simulink subsystem "Day3_Scenario_1"  (R2024a)
settings: Solver=VariableStepAuto  StartTime=0.0  StopTime=10.0  RelTol=1e-3
undefined symbols (not defined in the file): left_first_line_point_x, right_first_line_point_x
libraries: CarMaker4SL x6, slpidlib x1
settings Model: Creator=junhyung.cha  LastModifiedBy=junhyung.cha

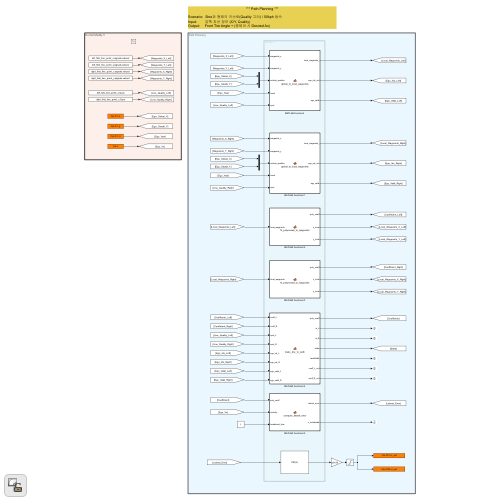
[thumbnail: Simulink's stored preview of the top-level diagram]
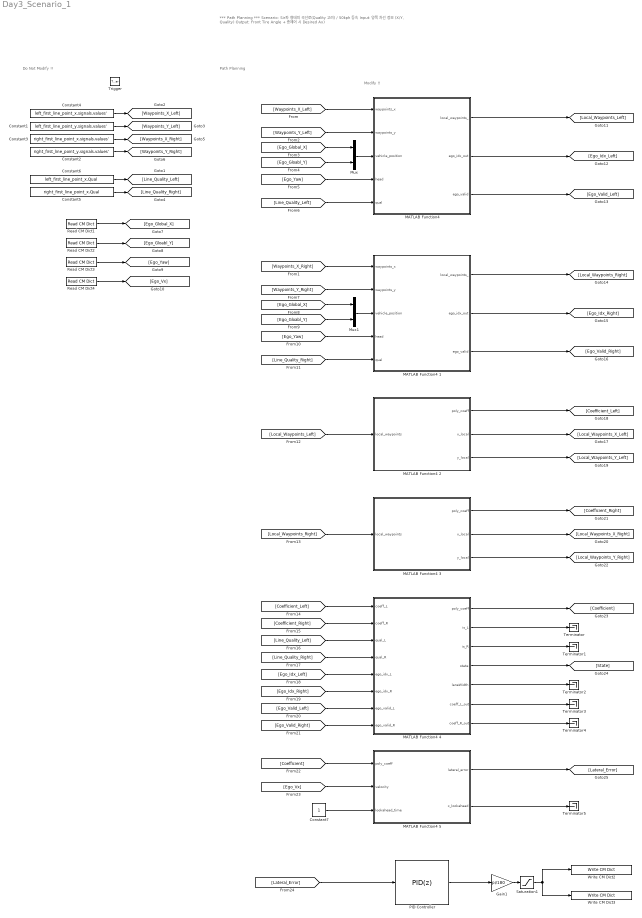
== system Day3_Scenario_1 ==
  note: Path Planning
  note: Do Not Modify !!
  note: Modify !!
  note: *** Path Planning ***
      |
      | Scenario: Sine파 형태의 곡선로(Quality 고려) / 50kph 등속
      | Input: 양쪽 차선 정보 (X/Y, Quality)
      | Output: Front Tire Angle + (종제어 시 Desired Ax)
  Trigger : TriggerPort  TriggerType=function-call  VariantControl=(inherit)
  Constant1 : Constant  Value=left_first_line_point_y.signals.values'
  Constant2 : Constant  Value=right_first_line_point_y.signals.values'
  Constant3 : Constant  Value=right_first_line_point_x.signals.values'
  Constant4 : Constant  Value=left_first_line_point_x.signals.values'
  Constant5 : Constant  Value=right_first_line_point_x.Qual
  Constant6 : Constant  Value=left_first_line_point_x.Qual
  Constant7 : Constant
  Gain1 : Gain  Gain=pi/180
  "MATLAB Function4 " : MATLAB Function  TreatAsAtomicUnit=on
  MATLAB Function4 1 : MATLAB Function  TreatAsAtomicUnit=on
  MATLAB Function4 2 : MATLAB Function  TreatAsAtomicUnit=on
  MATLAB Function4 3 : MATLAB Function  TreatAsAtomicUnit=on
  MATLAB Function4 4 : MATLAB Function  TreatAsAtomicUnit=on
  MATLAB Function4 5 : MATLAB Function  TreatAsAtomicUnit=on
  Mux : Mux  Inputs=2
  Mux1 : Mux  Inputs=2
  PID Controller : slpidlib/PID Controller  Controller=PID  Form=Parallel  TimeDomain=Discrete-time  UseExternalTs=off  SampleTime=-1  IntegratorMethod=Forward Euler  FilterMethod=Forward Euler  ControllerParametersSource=internal  P=3  I=0.01  UseKiTs=off  D=0  UseExternalDerivativeSource=off  N=100  UseFilter=on  TunerSelectOption=Transfer Function Based (PID Tuner App)  InitialConditionSource=internal  InitialConditionForIntegrator=0  InitialConditionForFilter=0  DifferentiatorICPrevScaledInput=0  ExternalReset=none  TrackingMode=off  Kt=1  LimitOutput=off  SatLimitsSource=internal  UpperSaturationLimit=inf  LowerSaturationLimit=-inf  LinearizeAsGain=on  AntiWindupMode=none  Kb=1  LimitIntegrator=off  UpperIntegratorSaturationLimit=inf  LowerIntegratorSaturationLimit=-inf  POutMin=[]  POutMax=[]  IOutMin=[]  IOutMax=[]  DOutMin=[]  DOutMax=[]  NOutMin=[]  NOutMax=[]  SumOutMin=[]  SumOutMax=[]  SaturationOutMin=[]  SaturationOutMax=[]  PParamMin=[]  PParamMax=[]  IParamMin=[]  IParamMax=[]  DParamMin=[]  DParamMax=[]  NParamMin=[]  NParamMax=[]  KbParamMin=[]  KbParamMax=[]  KtParamMin=[]  KtParamMax=[]  KbOutMin=[]  KbOutMax=[]  KtOutMin=[]  KtOutMax=[]  IntegratorOutMin=[]  IntegratorOutMax=[]  FilterOutMin=[]  FilterOutMax=[]  SumI1OutMin=[]  SumI1OutMax=[]  SumI2OutMin=[]  SumI2OutMax=[]  SumI3OutMin=[]  SumI3OutMax=[]  SumI4OutMin=[]  SumI4OutMax=[]  SumDOutMin=[]  SumDOutMax=[]  DifferentiatorOutMin=[]  DifferentiatorOutMax=[]  FilterDiffOutCoefMin=[]  FilterDiffOutCoefMax=[]  ReciprocalOutMin=[]  ReciprocalOutMax=[]  SumDenOutMin=[]  SumDenOutMax=[]  SumNumOutMin=[]  SumNumOutMax=[]  DivideOutMin=[]  DivideOutMax=[]  UdiffTsProdOutMin=[]  UdiffTsProdOutMax=[]  NTsProdOutMin=[]  NTsProdOutMax=[]  UintegralTsProdOutMin=[]  UintegralTsProdOutMax=[]  UngainTsProdOutMin=[]  UngainTsProdOutMax=[]  ClampingZeroOutDataTypeStr=Inherit: Inherit via back propagation  ClampingZeroOutMin=[]  ClampingZeroOutMax=[]  FilterDenConstantOutDataTypeStr=Inherit: Inherit via back propagation  FilterDenConstantOutMin=[]  FilterDenConstantOutMax=[]  PCopyOutDataTypeStr=Inherit: Inherit via back propagation  PCopyOutMin=[]  PCopyOutMax=[]  NCopyOutDataTypeStr=Inherit: Inherit via back propagation  NCopyOutMin=[]  NCopyOutMax=[]  IntegratorContinuousStateAttributes=''  IntegratorStateMustResolveToSignalObject=off  IntegratorRTWStateStorageClass=Auto  FilterContinuousStateAttributes=''  FilterStateMustResolveToSignalObject=off  FilterRTWStateStorageClass=Auto  ParallelPVariant=InternalParameters  IdealPVariant=Disabled  IVariant=InternalParameters  DVariant=InternalParameters  IntegratorVariant=Discrete  SatVariant=Disabled  AWVariant=Passthrough  PCopyVariant=Disabled  TRVariant=Disabled  FdbkBlocksVariant=Forward  IdealPFdbkVariant=Disabled  SatFdbkVariant=Disabled  DerivativeFilterVariant=ForwardEulerFilter  NVariant=InternalParameters  NCopyVariant=Disabled  FilterICVariant=InternalICsFilter  IntegratorICVariant=InternalICs  ExternalResetVariant=Disabled  TRSumVariant=Passthrough  SumFdbkVariant=Disabled  SumVariant=Sum_PID  TsampFilterVariant=InternalTs  TsampNgainVariant=Passthrough  TsampIntegralVariant=Disabled_SignalSpec  ExternalSaturationOutDataTypeStr=Inherit: Same as second input  DerivativeSourceVariant=ErrorSignal
  Read CM Dict1 : CarMaker4SL/Read CM Dict  xname=Car.Fr1.tx  xsync=off  xstime=Inherited
  Read CM Dict2 : CarMaker4SL/Read CM Dict  xname=Car.Fr1.ty  xsync=off  xstime=Inherited
  Read CM Dict3 : CarMaker4SL/Read CM Dict  xname=Car.Fr1.rz  xsync=off  xstime=Inherited
  Read CM Dict4 : CarMaker4SL/Read CM Dict  xname=Car.v  xsync=off  xstime=Inherited
  Saturation1 : Saturate  UpperLimit=2  LowerLimit=-2
  Terminator{,1..5} (6 alike) : Terminator
  Write CM Dict2 : CarMaker4SL/Write CM Dict  xname=Car.CFL.rz_ext  xsync=off
  Write CM Dict3 : CarMaker4SL/Write CM Dict  xname=Car.CFR.rz_ext  xsync=off
  wires:
  Constant4/1 -> [Waypoints_X_Left]
  Constant1/1 -> [Waypoints_Y_Left]
  Constant2/1 -> [Waypoints_Y_Right]
  Constant3/1 -> [Waypoints_X_Right]
  [Waypoints_X_Left] -> "MATLAB Function4 "/1(waypoints_x)
  [Waypoints_Y_Left] -> "MATLAB Function4 "/2(waypoints_y)
  Mux/1 -> "MATLAB Function4 "/3(vehicle_position)
  [Ego_Global_X] -> Mux/1
  Read CM Dict2/1 -> [Ego_Gloabl_Y]
  Read CM Dict1/1 -> [Ego_Global_X]
  [Ego_Gloabl_Y] -> Mux/2
  Read CM Dict3/1 -> [Ego_Yaw]
  [Ego_Yaw] -> "MATLAB Function4 "/4(head)
  Constant5/1 -> [Line_Quality_Right]
  Constant6/1 -> [Line_Quality_Left]
  [Line_Quality_Left] -> "MATLAB Function4 "/5(qual)
  [Line_Quality_Right] -> MATLAB Function4 1/5(qual)
  [Ego_Yaw] -> MATLAB Function4 1/4(head)
  [Ego_Gloabl_Y] -> Mux1/2
  [Ego_Global_X] -> Mux1/1
  [Waypoints_Y_Right] -> MATLAB Function4 1/2(waypoints_y)
  [Waypoints_X_Right] -> MATLAB Function4 1/1(waypoints_x)
  Mux1/1 -> MATLAB Function4 1/3(vehicle_position)
  "MATLAB Function4 "/3(ego_valid) -> [Ego_Valid_Left]
  "MATLAB Function4 "/2(ego_idx_out) -> [Ego_Idx_Left]
  "MATLAB Function4 "/1(local_waypoints_) -> [Local_Waypoints_Left]
  MATLAB Function4 1/1(local_waypoints_) -> [Local_Waypoints_Right]
  MATLAB Function4 1/2(ego_idx_out) -> [Ego_Idx_Right]
  MATLAB Function4 1/3(ego_valid) -> [Ego_Valid_Right]
  [Local_Waypoints_Left] -> MATLAB Function4 2/1(local_waypoints)
  [Local_Waypoints_Right] -> MATLAB Function4 3/1(local_waypoints)
  MATLAB Function4 2/1(poly_coeff) -> [Coefficient_Left]
  MATLAB Function4 2/2(x_local) -> [Local_Waypoints_X_Left]
  MATLAB Function4 2/3(y_local) -> [Local_Waypoints_Y_Left]
  MATLAB Function4 3/3(y_local) -> [Local_Waypoints_Y_Right]
  MATLAB Function4 3/2(x_local) -> [Local_Waypoints_X_Right]
  MATLAB Function4 3/1(poly_coeff) -> [Coefficient_Right]
  [Coefficient_Left] -> MATLAB Function4 4/1(coeff_L)
  [Coefficient_Right] -> MATLAB Function4 4/2(coeff_R)
  [Line_Quality_Left] -> MATLAB Function4 4/3(qual_L)
  [Line_Quality_Right] -> MATLAB Function4 4/4(qual_R)
  [Ego_Idx_Left] -> MATLAB Function4 4/5(ego_idx_L)
  [Ego_Idx_Right] -> MATLAB Function4 4/6(ego_idx_R)
  [Ego_Valid_Left] -> MATLAB Function4 4/7(ego_valid_L)
  [Ego_Valid_Right] -> MATLAB Function4 4/8(ego_valid_R)
  MATLAB Function4 4/1(poly_coeff) -> [Coefficient]
  MATLAB Function4 4/4(state) -> [State]
  MATLAB Function4 4/2(is_L) -> Terminator/1
  MATLAB Function4 4/3(is_R) -> Terminator1/1
  MATLAB Function4 4/6(coeff_L_out) -> Terminator3/1
  MATLAB Function4 4/5(laneWidth) -> Terminator2/1
  MATLAB Function4 4/7(coeff_R_out) -> Terminator4/1
  [Coefficient] -> MATLAB Function4 5/1(poly_coeff)
  Read CM Dict4/1 -> [Ego_Vx]
  [Ego_Vx] -> MATLAB Function4 5/2(velocity)
  Constant7/1 -> MATLAB Function4 5/3(lookahead_time)
  Saturation1/1 -> Write CM Dict3/1, Write CM Dict2/1
  Gain1/1 -> Saturation1/1
  MATLAB Function4 5/1(lateral_error) -> [Lateral_Error]
  MATLAB Function4 5/2(x_lookahead) -> Terminator5/1
  [Lateral_Error] -> PID Controller/1
  PID Controller/1 -> Gain1/1

== matlab function Day3_Scenario_1/MATLAB Function4  ==
  settings: sampleTime=0.1
  data: waypoints_x input; waypoints_y input; local_waypoints_ output; vehicle_position input; head input; qual input; ego_idx_out output; ego_valid output
function [local_waypoints_,ego_idx_out,ego_valid]  = global_to_local_waypoints(waypoints_x,waypoints_y, vehicle_position, head, qual)
    [local_waypoints_,ego_idx_out,ego_valid] = deal(0);
end

== matlab function Day3_Scenario_1/MATLAB Function4 1 ==
  settings: sampleTime=0.1
  data: waypoints_x input; waypoints_y input; local_waypoints_ output; vehicle_position input; head input; qual input; ego_idx_out output; ego_valid output
function [local_waypoints_,ego_idx_out,ego_valid]  = global_to_local_waypoints(waypoints_x,waypoints_y, vehicle_position, head, qual)
    [local_waypoints_,ego_idx_out,ego_valid] = deal(0);
end

== matlab function Day3_Scenario_1/MATLAB Function4 2 ==
  settings: sampleTime=0.1
  data: local_waypoints input; poly_coeff output; x_local output; y_local output
function [poly_coeff,x_local,y_local] = fit_polynomial_to_waypoints(local_waypoints)
    [poly_coeff,x_local,y_local] = deal(0);
end

== matlab function Day3_Scenario_1/MATLAB Function4 3 ==
  settings: sampleTime=0.1
  data: local_waypoints input; poly_coeff output; x_local output; y_local output
function [poly_coeff,x_local,y_local] = fit_polynomial_to_waypoints(local_waypoints)
    [poly_coeff,x_local,y_local] = deal(0);
end

== matlab function Day3_Scenario_1/MATLAB Function4 4 ==
  settings: sampleTime=0.1
  data: coeff_L input; poly_coeff output; is_L output; is_R output; coeff_R input; qual_L input; qual_R input; ego_idx_L input; ego_idx_R input; ego_valid_L input; ego_valid_R input; state output; laneWidth output; coeff_L_out output; coeff_R_out output
function [poly_coeff,is_L,is_R,state,laneWidth,coeff_L_out,coeff_R_out] = make_line_to_path(coeff_L,coeff_R,qual_L,qual_R,ego_idx_L, ego_idx_R,ego_valid_L,ego_valid_R)
    [poly_coeff,is_L,is_R,state,laneWidth,coeff_L_out,coeff_R_out] = deal(0);
end

== matlab function Day3_Scenario_1/MATLAB Function4 5 ==
  settings: sampleTime=0.1
  data: poly_coeff input; lateral_error output; x_lookahead output; velocity input; lookahead_time input
function [lateral_error,x_lookahead] = compute_lateral_error(poly_coeff, velocity, lookahead_time)
    [lateral_error,x_lookahead] = deal(0);
end
